simulink model "qbmove_example"  (R2016a)
settings: Solver=ode1  StartTime=0.0  StopTime=inf  FixedStep=.0005  RelTol=1e-3
libraries: qbmove_library x5, QB_pacer_lib x1
settings Model: Creator=laurentio  LastModifiedBy=MattiaCP
settings DataIOCC: LimitDataPoints=on  SaveFormat=Array
settings DebuggingCC: UnderspecifiedInitializationDetection=Classic  MergeDetectMultiDrivingBlocksExec=none  SolverPrmCheckMsg=warning  AllowSymbolicDim=off  StateNameClashWarn=warning
settings HardwareCC: ProdBitPerPointer=32  ProdLargestAtomicFloat=None  ProdIntDivRoundTo=Undefined  ProdEndianess=Unspecified  ProdWordSize=32  ProdHWDeviceType=32-bit Generic
settings ModelReferenceCC: PropagateSignalLabelsOutOfModel=off
settings ConfigComp: CovModelRefEnable=Off  CovSFcnEnable=off

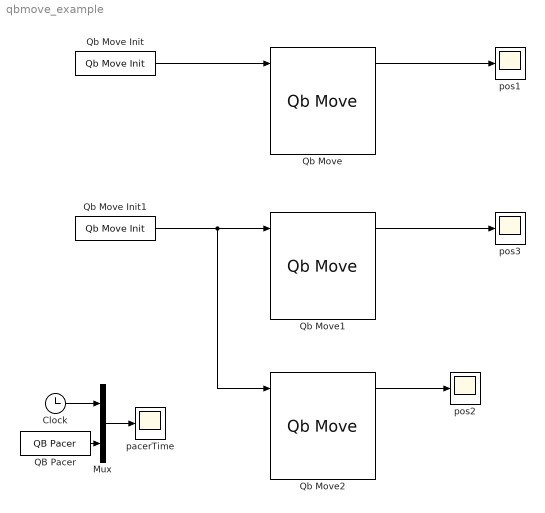
== system qbmove_example ==
  Clock : Clock
  Mux : Mux  Inputs=2
  QB Pacer : QB_pacer_lib/QB Pacer  simTimePerRealTime=1
  Qb Move : qbmove_library/Qb Move  ID=1  ACTIVE_COMM_DIRECTIONS=Both  CONTROL_MODE=Prime Movers Positions  DAISY_CHAINING=off  MAX_ANG=0  SW_LIMIT=inf  OFFSET=0  ACTIVATE=off  WDT=0.0  UNIT=Degrees
  Qb Move Init : qbmove_library/Qb Move Init  NUMBER_OF_COM='COM12'  BAUD_RATE_COM=2000000
  Qb Move Init1 : qbmove_library/Qb Move Init  NUMBER_OF_COM='COM19'  BAUD_RATE_COM=2000000
  Qb Move1 : qbmove_library/Qb Move  ID=2  ACTIVE_COMM_DIRECTIONS=Both  CONTROL_MODE=Prime Movers Positions  DAISY_CHAINING=off  MAX_ANG=0  SW_LIMIT=inf  OFFSET=0  ACTIVATE=off  WDT=0.0  UNIT=Degrees
  Qb Move2 : qbmove_library/Qb Move  ID=1  ACTIVE_COMM_DIRECTIONS=Both  CONTROL_MODE=Prime Movers Positions  DAISY_CHAINING=off  MAX_ANG=0  SW_LIMIT=inf  OFFSET=0  ACTIVATE=off  WDT=0.0  UNIT=Degrees
  pacerTime : Scope
  pos1 : Scope
  pos2 : Scope
  pos3 : Scope
  wires:
  QB Pacer/1 -> Mux/2
  Clock/1 -> Mux/1
  Qb Move Init/1 -> Qb Move/1
  Mux/1 -> pacerTime/1
  Qb Move/1 -> pos1/1
  Qb Move Init1/1 -> Qb Move2/1, Qb Move1/1
  Qb Move1/1 -> pos3/1
  Qb Move2/1 -> pos2/1
